simulink model "bluetooth_voice"  (Simulink 4.1.1)
settings: Solver=VariableStepDiscrete  StartTime=0.0  StopTime=2.7  RelTol=1e-3
PreLoadFcn:
  | bluetooth_init;
values from neighbouring files (symbols this model uses):
  Access_Code = zeros(72,1); Access_Code(1:2:72)=1    [bluetooth_init.m]
  ARQ = [1]    [bluetooth_init.m]
  awgn_channel_seed = randseed(2)    [bluetooth_init.m]
  data_seed = randseed(5)    [bluetooth_init.m]
  Flow_Control = [1]    [bluetooth_init.m]
  Input_Fs = 8000    [bluetooth_init.m]
  Num_Slots_Rate = 6    [device_init.m]
  One_Zero_Payload = zeros(240,1)    [bluetooth_init.m]
  Packet_Type = [1 0 1 0]'    [bluetooth_init.m]
  Sequence = [1]    [bluetooth_init.m]
  Slave_Address = [1 0 1]'    [bluetooth_init.m]
  Slot_Enable_Phase = Slot_Pair*2-2    [device_init.m]
  Slot_Ts = (1/1600)    (= 0.000625)    [device_init.m]
  Tx_Ts = Slot_Ts*6    (= 0.00375)    [device_init.m]
undefined symbols (not defined in the file or in its folder): Fs, g, jet
libraries: commblkcod2 x48, dspsrcs3 x25, dspsigops x18, simulink3 x16, dspsigattribs x9, dspbuff3 x7, dspindex x7, bluetooth_lib x5, dspmathops x4, dspsnks3 x4, dspmtrx3 x3, commdigbbndfm2 x3
(part 2 of 2)

== system bluetooth_voice/Slave Receiver/Demodulate and decode/GMSK Demodulate and frequency hop ==
  Rx Signal : Inport  Port=1  LatchInput=off
  Hop : Inport  Port=2  LatchInput=off
  Extract 366 bits with one symbol delay : Selector  InputType=Vector  ElementSrc=Internal  Elements=[2:367]  RowSrc=Internal  Rows=1  ColumnSrc=Internal  Columns=1  InputPortWidth=625
  Frame Status Conversion : dspsigattribs/Frame Status Conversion  growRefPort=off  outframe=Frame-based
  "Generate 79 possible carriers -39MHz to 39MHz " : commdigbbndfm2/M-FSK Modulator Baseband  M=79  InType=Integer  Enc=Binary  freqSep=1e6  phaseType=Continuous  numSamp=6.25e4
  IF Filter Select 1MHz band1 : dsparch3/Digital Filter Design
  M-FSK Demodulator Baseband : commdigbbndfm2/M-FSK Demodulator Baseband  M=2  OutType=Bit  Dec=Binary  freqSep=2*150e3  numSamp=100
  Math Function : Math  Orientation=up  Operator=conj  OutputSignalType=auto
  Move to a symbol boundary : dspsigops/Integer Delay  delay=100-50  ic=0
  Product1 : Product  Inputs=2  Multiplication=Element-wise(.*)  SaturateOnIntegerOverflow=on
  Rx Raw Bits : Outport  Port=1
  wires:
  Move to a symbol boundary/1 -> M-FSK Demodulator Baseband/1
  IF Filter Select 1MHz band1/1 -> Move to a symbol boundary/1
  Frame Status Conversion/1 -> "Generate 79 possible carriers -39MHz to 39MHz "/1
  "Generate 79 possible carriers -39MHz to 39MHz "/1 -> Math Function/1
  Math Function/1 -> Product1/2
  Product1/1 -> IF Filter Select 1MHz band1/1
  M-FSK Demodulator Baseband/1 -> Extract 366 bits with one symbol delay/1
  Rx Signal/1 -> Product1/1
  Extract 366 bits with one symbol delay/1 -> Rx Raw Bits/1
  Hop/1 -> Frame Status Conversion/1

== system bluetooth_voice/Slave Receiver/Demodulate and decode/HEC Fail ==
  In : Inport  Port=1  LatchInput=off
  Any HEC bits not matching : Logic  Operator=OR  Inputs=1
  Bluetooth HEC Generator1 : Subsystem  mask(Bluetooth HEC Generator){uap=[1 0 0 1 0 1 1 0]}
      mask help: Compute the Bluetooth Header Error Check (HEC) as specified in section 5.4 of the Bluetooth specification. The Upper Address Part (UAP) is used to initialize the state of the encoder. The UAP is an 8-bit vector, LSB first.
      settings: RTWFcnNameOpts=Auto  RTWFileNameOpts=Auto
      mask Display: disp('Bluetooth\nHEC Generator')
  Demux : Demux  Outputs=[10 8]  BusSelectionMode=off
  Relational Operator1 : RelationalOperator  Operator=~=
  Out : Outport  Port=1
  wires:
  Any HEC bits not matching/1 -> Out/1
  In/1 -> Demux/1
  Bluetooth HEC Generator1/1(Out1) -> Relational Operator1/1
  Demux/2 -> Relational Operator1/2
  Demux/1 -> Bluetooth HEC Generator1/1(In1)
  Relational Operator1/1 -> Any HEC bits not matching/1

== system bluetooth_voice/Slave Receiver/Demodulate and decode/Header info FEC Decode ==
  In : Inport  Port=1  LatchInput=off
  Constant1 : Constant  Value=.5
  Decode FEC : commsequence2/Derepeat  N=3  ic=0  mode=Maintain input frame rate
  Threshold : RelationalOperator  Operator=>
  Out : Outport  Port=1
  wires:
  Threshold/1 -> Out/1  "HEC"
  In/1 -> Decode FEC/1
  Decode FEC/1 -> Threshold/1
  Constant1/1 -> Threshold/2

== system bluetooth_voice/Slave Receiver/Demodulate and decode/One Zeros ==
  Constant : Constant  Value=HV_Type
  FEC HV1 : Subsystem  TreatAsAtomicUnit=on
      settings: RTWFcnNameOpts=Auto  RTWFileNameOpts=Auto
  FEC HV2 : Subsystem  TreatAsAtomicUnit=on
      settings: RTWFcnNameOpts=Auto  RTWFileNameOpts=Auto
  FEC HV3 (None) : Subsystem  TreatAsAtomicUnit=on
      settings: RTWFcnNameOpts=Auto  RTWFileNameOpts=Auto
  Fcn : Fcn  Expr=u==1
  Fcn1 : Fcn  Expr=u==2
  Fcn2 : Fcn  Expr=u==3
  Merge : Merge  Inputs=3  AllowUnequalInputPortWidths=off  InputPortOffsets=[]
  One Zeros : Outport  Port=1
  wires:
  Constant/1 -> Fcn/1, Fcn1/1, Fcn2/1
  Fcn/1 -> FEC HV1/Enable
  Fcn1/1 -> FEC HV2/Enable
  Fcn2/1 -> FEC HV3 (None)/Enable
  FEC HV2/1(Ones Zeros) -> Merge/2
  FEC HV1/1(Ones Zeros) -> Merge/1
  Merge/1 -> One Zeros/1
  FEC HV3 (None)/1(Ones Zeros) -> Merge/3

== system bluetooth_voice/Slave Receiver/Demodulate and decode/Payload FEC Decode ==
  Input Bits : Inport  Port=1  LatchInput=off
  Constant : Constant  Value=HV_Type
  FEC HV1 : Subsystem  TreatAsAtomicUnit=on
      settings: RTWFcnNameOpts=Auto  RTWFileNameOpts=Auto
  FEC HV2 : Subsystem  TreatAsAtomicUnit=on
      settings: RTWFcnNameOpts=Auto  RTWFileNameOpts=Auto
  FEC HV3 (None) : Subsystem  TreatAsAtomicUnit=on
      settings: RTWFcnNameOpts=Auto  RTWFileNameOpts=Auto
  Fcn : Fcn  Expr=u==1
  Fcn1 : Fcn  Expr=u==2
  Fcn2 : Fcn  Expr=u==3
  Merge : Merge  Inputs=3  AllowUnequalInputPortWidths=off  InputPortOffsets=[]
  Payload Bits1 : dspindex/Multiport Selector  rowsOrCols=Rows  idxCellArray={1:Num_Payload_Bits}  idxErrMode=Clip Index
  Decoded Bits : Outport  Port=1
  wires:
  Payload Bits1/1 -> Decoded Bits/1
  Merge/1 -> Payload Bits1/1
  FEC HV3 (None)/1(FEC'd) -> Merge/3
  FEC HV1/1(FEC'd) -> Merge/1
  FEC HV2/1(FEC'd) -> Merge/2
  Fcn2/1 -> FEC HV3 (None)/Enable
  Fcn1/1 -> FEC HV2/Enable
  Fcn/1 -> FEC HV1/Enable
  Constant/1 -> Fcn1/1, Fcn2/1, Fcn/1
  Input Bits/1 -> FEC HV1/1(In), FEC HV2/1(In), FEC HV3 (None)/1(In)

== system bluetooth_voice/Slave Receiver/Demodulate and decode/Residual BER Subsystem ==
  In1 : Inport  Port=1  LatchInput=off
  In2 : Inport  Port=2  LatchInput=off
  Enable : EnablePort
  Residual BER : commsink2/Error Rate Calculation  N=0  st_delay=0  cp_mode=Entire frame  subframe=[]  PMode=Port  WsName=ErrorVec  RsMode2=off  stop=off  numErr=100  maxBits=1e6
  Out1 : Outport  Port=1
  wires:
  In2/1 -> Residual BER/2
  Residual BER/1 -> Out1/1
  In1/1 -> Residual BER/1

== system bluetooth_voice/Master Transmitter/CVSD Encode/Set any 0's to 1's/Pass through ==
  In1 : Inport  Port=1  LatchInput=off
  Action Port : ActionPort  InitializeStates=held  ActionType=else
  Out1=In1 : Outport  Port=1
  wires:
  In1/1 -> Out1=In1/1

== system bluetooth_voice/Master Transmitter/CVSD Encode/Set any 0's to 1's/Set to 1 ==
  Action Port : ActionPort  InitializeStates=held  ActionType=then
  DSP Constant : dspsrcs3/DSP Constant  Value=1  InterpretAs1D=on  SampleMode=Discrete  Ts=1/64000  FramebasedOutput=off
  1 : Outport  Port=1
  wires:
  DSP Constant/1 -> 1/1

== system bluetooth_voice/Master Transmitter/CVSD Encode/Update stepsize/Update ==
  stepsize : Inport  Port=1  LatchInput=off
  Action Port : ActionPort  InitializeStates=held  ActionType=then
  Constant : Constant  Value=min_step
  Constant1 : Constant  Value=max_step
  MinMax : MinMax  Function=min  Inputs=2
  Sum2 : Sum  Inputs=|++  SaturateOnIntegerOverflow=on
  stepsize(n+1) : Outport  Port=1
  wires:
  Constant/1 -> Sum2/1
  Sum2/1 -> MinMax/1
  Constant1/1 -> MinMax/2
  MinMax/1 -> stepsize(n+1)/1
  stepsize/1 -> Sum2/2

== system bluetooth_voice/Master Transmitter/CVSD Encode/Update stepsize/Update1 ==
  stepsize : Inport  Port=1  LatchInput=off
  Action Port : ActionPort  InitializeStates=held  ActionType=else
  Constant1 : Constant  Value=min_step
  Gain : Gain  Gain=step_decay  Multiplication=Element-wise(K.*u)  SaturateOnIntegerOverflow=on
  MinMax : MinMax  Function=max  Inputs=2
  stepsize(n+1) : Outport  Port=1
  wires:
  MinMax/1 -> stepsize(n+1)/1
  Constant1/1 -> MinMax/2
  Gain/1 -> MinMax/1
  stepsize/1 -> Gain/1

== system bluetooth_voice/Slave Receiver/CVSD Decode/Update stepsize/Update ==
  stepsize : Inport  Port=1  LatchInput=off
  Action Port : ActionPort  InitializeStates=held  ActionType=then
  Constant : Constant  Value=min_step
  Constant1 : Constant  Value=max_step
  MinMax : MinMax  Function=min  Inputs=2
  Sum2 : Sum  Inputs=|++  SaturateOnIntegerOverflow=on
  stepsize(n+1) : Outport  Port=1
  wires:
  Constant/1 -> Sum2/1
  Sum2/1 -> MinMax/1
  Constant1/1 -> MinMax/2
  MinMax/1 -> stepsize(n+1)/1
  stepsize/1 -> Sum2/2

== system bluetooth_voice/Slave Receiver/CVSD Decode/Update stepsize/Update1 ==
  stepsize : Inport  Port=1  LatchInput=off
  Action Port : ActionPort  InitializeStates=held  ActionType=else
  Constant1 : Constant  Value=min_step
  Gain : Gain  Gain=step_decay  Multiplication=Element-wise(K.*u)  SaturateOnIntegerOverflow=on
  MinMax : MinMax  Function=max  Inputs=2
  stepsize(n+1) : Outport  Port=1
  wires:
  MinMax/1 -> stepsize(n+1)/1
  Constant1/1 -> MinMax/2
  Gain/1 -> MinMax/1
  stepsize/1 -> Gain/1

== system bluetooth_voice/Slave Receiver/Demodulate and decode/HEC Fail/Bluetooth HEC Generator1 ==
  In1 : Inport  Port=1  LatchInput=off
  Frame Status Conversion : dspsigattribs/Frame Status Conversion  growRefPort=off  outframe=Sample-based
  Frame Status Conversion1 : dspsigattribs/Frame Status Conversion  growRefPort=on  outframe=Sample-based
  S-Function Builder : S-Function  AncestorBlock=|  FunctionName=scomdemohecgen  Parameters=uap  PortCounts=[]  SFunctionModules=scomdemohecgen_wrapper
      | simulink3/Functions
      | & Tables/Basic S-Function
      | Builder
      mask init:
      | val = [[.9  0.75 0.75 1 1 .9 .9 1]',[1 1 0.75 0.75 .9 .9 1 .9]'];
      | sys = get_param(gcb,'FunctionName');
      settings: CopyFcn=set_param(gcb,'LinkStatus','none')  OpenFcn=sfunctionwizard(gcbh)
      mask Display:
      | plot(val(:,1),val(:,2))
      | disp(sys)
  Out1 : Outport  Port=1
  wires:
  S-Function Builder/1 -> Frame Status Conversion1/1
  In1/1 -> Frame Status Conversion/1, Frame Status Conversion1/2
  Frame Status Conversion1/1 -> Out1/1
  Frame Status Conversion/1 -> S-Function Builder/1

== system bluetooth_voice/Slave Receiver/Demodulate and decode/One Zeros/FEC HV1 ==
  Enable : EnablePort
  1 0 1 0 1 0 ... : dspsrcs3/DSP Constant  Value=One_Zero_Payload(1:80)  InterpretAs1D=off  SampleMode=Discrete  Ts=30*(1/Input_Fs)/6  FramebasedOutput=on
  FEC1 : dspsigops/Repeat  N=3  ic=0  mode=Maintain input frame rate
  Ones Zeros : Outport  Port=1
  wires:
  1 0 1 0 1 0 .../1 -> FEC1/1
  FEC1/1 -> Ones Zeros/1

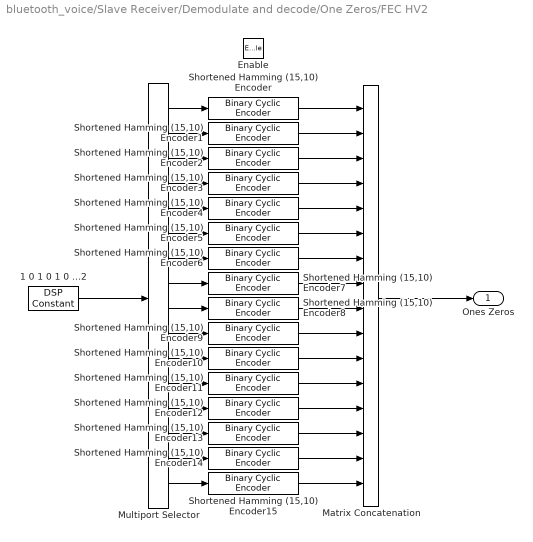
== system bluetooth_voice/Slave Receiver/Demodulate and decode/One Zeros/FEC HV2 ==
  Enable : EnablePort
  1 0 1 0 1 0 ...2 : dspsrcs3/DSP Constant  Value=One_Zero_Payload(1:160)  InterpretAs1D=off  SampleMode=Discrete  Ts=Slot_Ts  FramebasedOutput=on
  Matrix Concatenation : simulink3/Signals & Systems/Matrix Concatenation  numInports=16  catMethod=Vertical
  Multiport Selector : dspindex/Multiport Selector  rowsOrCols=Rows  idxCellArray={ 1:10, 11:20,21:30,31:40,41:50,51:60,61:70,71:80,81:90,91:100,101:110,111:120,121:130,131:140,141:150,151:160}  idxErrMode=Clip Index
  Shortened Hamming (15,10) Encoder{,1..15} (16 alike) : commblkcod2/Binary Cyclic Encoder  n=15  p=[1 1 0 1 0 1]
  Ones Zeros : Outport  Port=1
  wires:
  1 0 1 0 1 0 ...2/1 -> Multiport Selector/1
  Multiport Selector/1 -> Shortened Hamming (15,10) Encoder/1
  Multiport Selector/2 -> Shortened Hamming (15,10) Encoder1/1
  Multiport Selector/3 -> Shortened Hamming (15,10) Encoder2/1
  Multiport Selector/4 -> Shortened Hamming (15,10) Encoder3/1
  Multiport Selector/5 -> Shortened Hamming (15,10) Encoder4/1
  Multiport Selector/6 -> Shortened Hamming (15,10) Encoder5/1
  Multiport Selector/7 -> Shortened Hamming (15,10) Encoder6/1
  Multiport Selector/8 -> Shortened Hamming (15,10) Encoder7/1
  Multiport Selector/9 -> Shortened Hamming (15,10) Encoder8/1
  Multiport Selector/10 -> Shortened Hamming (15,10) Encoder9/1
  Multiport Selector/11 -> Shortened Hamming (15,10) Encoder10/1
  Multiport Selector/12 -> Shortened Hamming (15,10) Encoder11/1
  Multiport Selector/13 -> Shortened Hamming (15,10) Encoder12/1
  Multiport Selector/14 -> Shortened Hamming (15,10) Encoder13/1
  Multiport Selector/15 -> Shortened Hamming (15,10) Encoder14/1
  Multiport Selector/16 -> Shortened Hamming (15,10) Encoder15/1
  Shortened Hamming (15,10) Encoder/1 -> Matrix Concatenation/1
  Shortened Hamming (15,10) Encoder1/1 -> Matrix Concatenation/2
  Shortened Hamming (15,10) Encoder2/1 -> Matrix Concatenation/3
  Shortened Hamming (15,10) Encoder3/1 -> Matrix Concatenation/4
  Shortened Hamming (15,10) Encoder4/1 -> Matrix Concatenation/5
  Shortened Hamming (15,10) Encoder5/1 -> Matrix Concatenation/6
  Shortened Hamming (15,10) Encoder6/1 -> Matrix Concatenation/7
  Shortened Hamming (15,10) Encoder7/1 -> Matrix Concatenation/8
  Shortened Hamming (15,10) Encoder8/1 -> Matrix Concatenation/9
  Shortened Hamming (15,10) Encoder9/1 -> Matrix Concatenation/10
  Shortened Hamming (15,10) Encoder10/1 -> Matrix Concatenation/11
  Shortened Hamming (15,10) Encoder11/1 -> Matrix Concatenation/12
  Shortened Hamming (15,10) Encoder12/1 -> Matrix Concatenation/13
  Shortened Hamming (15,10) Encoder13/1 -> Matrix Concatenation/14
  Shortened Hamming (15,10) Encoder14/1 -> Matrix Concatenation/15
  Shortened Hamming (15,10) Encoder15/1 -> Matrix Concatenation/16
  Matrix Concatenation/1 -> Ones Zeros/1

== system bluetooth_voice/Slave Receiver/Demodulate and decode/One Zeros/FEC HV3 (None) ==
  Enable : EnablePort
  1 0 1 0 1 0 ... : dspsrcs3/DSP Constant  Value=One_Zero_Payload(1:240)  InterpretAs1D=off  SampleMode=Discrete  Ts=1/1600  FramebasedOutput=on
  Ones Zeros : Outport  Port=1
  wires:
  1 0 1 0 1 0 .../1 -> Ones Zeros/1

== system bluetooth_voice/Slave Receiver/Demodulate and decode/Payload FEC Decode/FEC HV1 ==
  In : Inport  Port=1  LatchInput=off
  Enable : EnablePort
  Constant1 : Constant  Value=.5
  Decode FEC : commsequence2/Derepeat  N=3  ic=One_Zero_Payload(1:80)  mode=Maintain input frame rate
  Threshold : RelationalOperator  Operator=>
  Zero Pad : dspsigops/Zero Pad  zpadAlong=Columns  numOutRows=240  numOutCols=1  trunc_flag=None
  FEC'd : Outport  Port=1
  wires:
  Zero Pad/1 -> FEC'd/1
  Decode FEC/1 -> Threshold/1
  Constant1/1 -> Threshold/2
  Threshold/1 -> Zero Pad/1
  In/1 -> Decode FEC/1

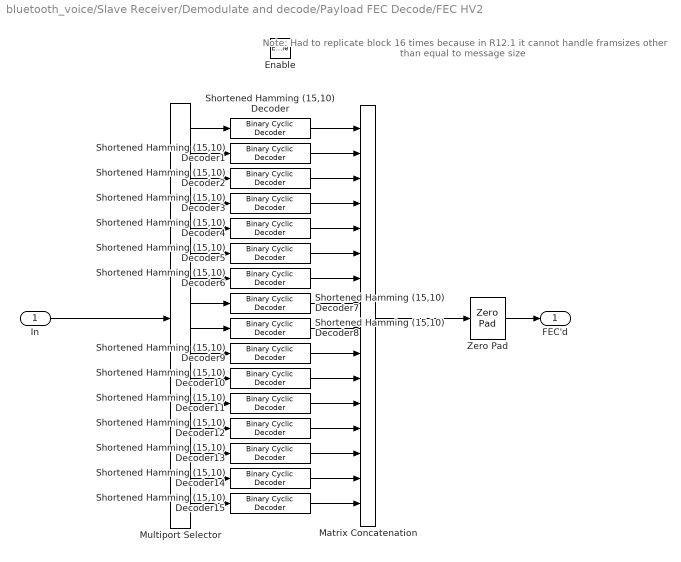
== system bluetooth_voice/Slave Receiver/Demodulate and decode/Payload FEC Decode/FEC HV2 ==
  note: Note: Had to replicate block 16 times
      | because in R12.1 it cannot handle framsizes
      | other than equal to message size
  In : Inport  Port=1  LatchInput=off
  Enable : EnablePort
  Matrix Concatenation : simulink3/Signals & Systems/Matrix Concatenation  numInports=16  catMethod=Vertical
  Multiport Selector : dspindex/Multiport Selector  rowsOrCols=Rows  idxCellArray={ 1:15, 16:30,31:45,46:60,61:75,76:90,91:105,106:120,121:135,136:150,151:165,166:180,181:195,196:210,211:225,226:240}  idxErrMode=Clip Index
  Shortened Hamming (15,10) Decoder{,1..15} (16 alike) : commblkcod2/Binary Cyclic Decoder  n=15  p=[1 1 0 1 0 1]
  Zero Pad : dspsigops/Zero Pad  zpadAlong=Columns  numOutRows=240  numOutCols=1  trunc_flag=None
  FEC'd : Outport  Port=1
  wires:
  Zero Pad/1 -> FEC'd/1
  Shortened Hamming (15,10) Decoder15/1 -> Matrix Concatenation/16
  Shortened Hamming (15,10) Decoder14/1 -> Matrix Concatenation/15
  Shortened Hamming (15,10) Decoder13/1 -> Matrix Concatenation/14
  Shortened Hamming (15,10) Decoder12/1 -> Matrix Concatenation/13
  Shortened Hamming (15,10) Decoder11/1 -> Matrix Concatenation/12
  Shortened Hamming (15,10) Decoder10/1 -> Matrix Concatenation/11
  Shortened Hamming (15,10) Decoder9/1 -> Matrix Concatenation/10
  Shortened Hamming (15,10) Decoder8/1 -> Matrix Concatenation/9
  Shortened Hamming (15,10) Decoder7/1 -> Matrix Concatenation/8
  Shortened Hamming (15,10) Decoder6/1 -> Matrix Concatenation/7
  Shortened Hamming (15,10) Decoder5/1 -> Matrix Concatenation/6
  Shortened Hamming (15,10) Decoder4/1 -> Matrix Concatenation/5
  Shortened Hamming (15,10) Decoder3/1 -> Matrix Concatenation/4
  Shortened Hamming (15,10) Decoder2/1 -> Matrix Concatenation/3
  Shortened Hamming (15,10) Decoder1/1 -> Matrix Concatenation/2
  Shortened Hamming (15,10) Decoder/1 -> Matrix Concatenation/1
  Matrix Concatenation/1 -> Zero Pad/1
  Multiport Selector/16 -> Shortened Hamming (15,10) Decoder15/1
  Multiport Selector/15 -> Shortened Hamming (15,10) Decoder14/1
  Multiport Selector/14 -> Shortened Hamming (15,10) Decoder13/1
  Multiport Selector/13 -> Shortened Hamming (15,10) Decoder12/1
  Multiport Selector/12 -> Shortened Hamming (15,10) Decoder11/1
  Multiport Selector/11 -> Shortened Hamming (15,10) Decoder10/1
  Multiport Selector/10 -> Shortened Hamming (15,10) Decoder9/1
  Multiport Selector/9 -> Shortened Hamming (15,10) Decoder8/1
  Multiport Selector/8 -> Shortened Hamming (15,10) Decoder7/1
  Multiport Selector/7 -> Shortened Hamming (15,10) Decoder6/1
  Multiport Selector/6 -> Shortened Hamming (15,10) Decoder5/1
  Multiport Selector/5 -> Shortened Hamming (15,10) Decoder4/1
  Multiport Selector/4 -> Shortened Hamming (15,10) Decoder3/1
  Multiport Selector/3 -> Shortened Hamming (15,10) Decoder2/1
  Multiport Selector/2 -> Shortened Hamming (15,10) Decoder1/1
  Multiport Selector/1 -> Shortened Hamming (15,10) Decoder/1
  In/1 -> Multiport Selector/1

== system bluetooth_voice/Slave Receiver/Demodulate and decode/Payload FEC Decode/FEC HV3 (None) ==
  In : Inport  Port=1  LatchInput=off
  Enable : EnablePort
  FEC'd : Outport  Port=1
  wires:
  In/1 -> FEC'd/1
